simulink model "example_model"  (R2018a)
settings: Solver=VariableStepAuto  StartTime=0.0  StopTime=10.0  RelTol=1e-3
undefined symbols (not defined in the file): DiscIntNeverNeededParam
settings Model: Creator=Yuxuan  LastModifiedBy=Yuxuan
settings DataIOCC: ReturnWorkspaceOutputs=on
settings DebuggingCC: UnconnectedInputMsg=none  UnconnectedOutputMsg=none  UnconnectedLineMsg=none  SFMachineParentedDataDiag=error
settings SFSimCC: SimUseLocalCustomCode=on
settings RTWCC: RTWUseLocalCustomCode=on

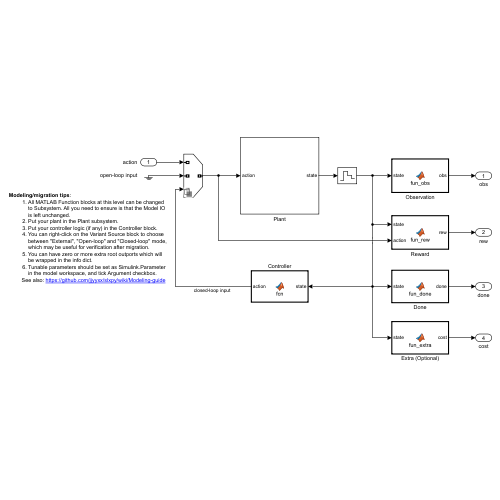
[thumbnail: Simulink's stored preview of the top-level diagram]
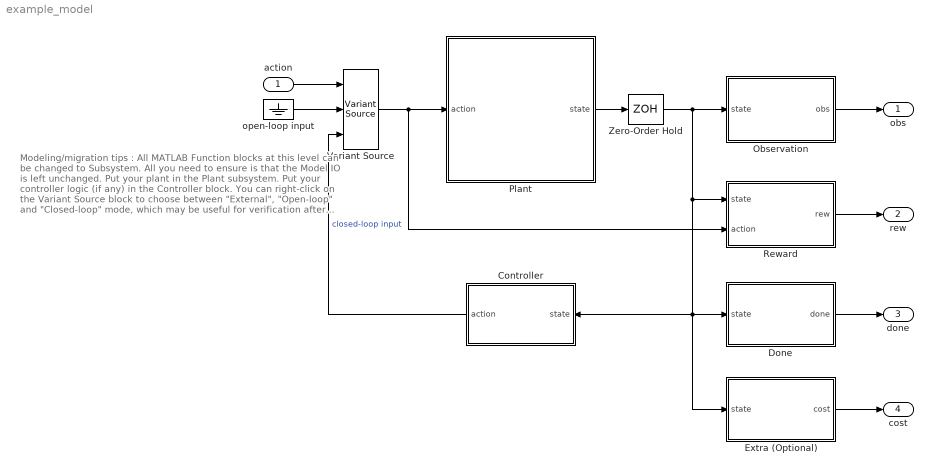
== system example_model ==
  note: Modeling/migration tips :
      | All MATLAB Function blocks at this level can be changed to Subsystem. All you need to ensure is that the Model IO is left unchanged.
      | Put your plant in the Plant subsystem.
      | Put your controller logic (if any) in the Controller block.
      | You can right-click on the Variant Source block to choose between "External", "Open-loop" and "Closed-loop" mode, which may be useful for verification after migration.
      | You can have zero or more extra root outports which will be wrapped in the info dict.
      | Tunable parameters should be set as Simulink.Parameter in the model workspace, and tick Argument checkbox.
      | See also: https://github.com/jjyyxx/slxpy/wiki/Modeling-guide
  action : Inport
  Controller : MATLAB Function  TreatAsAtomicUnit=on
  Done : MATLAB Function  TreatAsAtomicUnit=on
  Extra (Optional) : MATLAB Function  TreatAsAtomicUnit=on
  Observation : MATLAB Function  TreatAsAtomicUnit=on
  Plant : Subsystem
  Reward : MATLAB Function  TreatAsAtomicUnit=on
  Variant Source : VariantSource  OverrideUsingVariant=External
  Zero-Order Hold : ZeroOrderHold  SampleTime=-1
  open-loop input : Ground
  obs : Outport
  rew : Outport  Port=2
  done : Outport  Port=3
  cost : Outport  Port=4
  wires:
  Plant/1(state) -> Zero-Order Hold/1
  Variant Source/1 -> Reward/2(action), Plant/1(action)
  Observation/1(obs) -> obs/1
  Reward/1(rew) -> rew/1
  Done/1(done) -> done/1
  Zero-Order Hold/1 -> Observation/1(state), Controller/1(state), Extra (Optional)/1(state), Done/1(state), Reward/1(state)
  action/1 -> Variant Source/1
  open-loop input/1 -> Variant Source/2
  Controller/1(action) -> Variant Source/3  "closed-loop input"
  Extra (Optional)/1(cost) -> cost/1

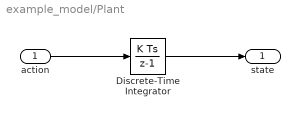
== system example_model/Plant ==
  action : Inport
  Discrete-Time Integrator : DiscreteIntegrator  SampleTime=-1  ICPrevOutput=DiscIntNeverNeededParam  ICPrevScaledInput=DiscIntNeverNeededParam
  state : Outport
  wires:
  action/1 -> Discrete-Time Integrator/1
  Discrete-Time Integrator/1 -> state/1

== matlab function example_model/Reward ==
  data: state input; rew output; action input
function rew = fun_rew(state, action)
rew = 0;

== matlab function example_model/Observation ==
  data: state input; obs output
function obs = fun_obs(state)
obs = state;

== matlab function example_model/Done ==
  data: state input; done output
function done = fun_done(state)
done = false;

== matlab function example_model/Controller ==
  data: state input; action output
function action = fcn(state)
action = -state;

== matlab function example_model/Extra (Optional) ==
  data: state input; cost output
function cost = fun_extra(state)
cost = 0.0;
